simulink model "AeropendulumSoftRTBangBang"  (Simulink 7.9)
settings: Solver=FixedStepDiscrete  SolverMode=SingleTasking  StartTime=0.0  StopTime=60  RelTol=1e-3
PreLoadFcn:
  | u0=21;
  | Slope=80;
  | Clag=1;
  | Clead=1;
  | clagd=1;
  | clead=1;
InitFcn:
  | out = instrfind;
  | delete(out);
  | s = serial('COM5');
  | set(s,'BaudRate',19200);
  | set(s,'InputBufferSize',2);
  | fopen(s);
StartFcn:
  | fwrite(s,128,'uchar');
StopFcn:
  | fclose(s)
undefined symbols (not defined in the file or in its folder): fread, fwrite
libraries: simulink x5, cstblocks x2
Description:
  | AeroPendulum Controller
  | -Phase lead
  | -Phase lag
  | -Proportional control
  | 
  | All controllers working!
settings Model: Creator=Josh Gill  LastModifiedBy=Enikov  ExtModeEnableFloating=off  ExtModeTrigDuration=10000  ExtModeLogAll=off
settings DataIOCC: SaveOutput=off  SignalLogging=off  DSMLogging=off  SaveTime=off
settings DebuggingCC: FcnCallInpInsideContextMsg=Use local settings  StrictBusMsg=Warning
settings HardwareCC: ProdIntDivRoundTo=Zero  ProdEndianess=LittleEndian  ProdHWDeviceType=Generic->32-bit x86 compatible
settings RTWCC: SystemTargetFile=rtwin.tlc  TemplateMakefile=rtwin.tmf  Description=Real-Time Windows Target  ProcessScript=rtwin_make_rtw_hook  RTWCompilerOptimization=On
settings CodeAppCC: MaxIdLength=95
settings RTWinTargetCC: TargetLibSuffix=_rtwin.lib  TargetPreCompLibLocation=C:\Program Files\MATLAB\R2012a\toolbox\rtw\targets\rtwin\lib\win64  CodeReplacementLibrary=ANSI_C  CodeExecutionProfiling=off  PortableWordSizes=off  RTWinDir=C:/PROGRA~1/MATLAB/R2012a/toolbox/rtw/targets/rtwin  TargetArch=win64

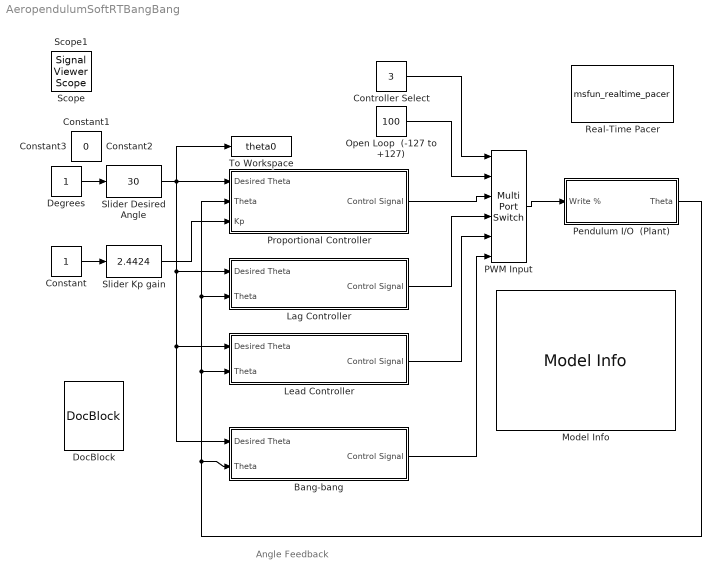
== system AeropendulumSoftRTBangBang ==
  note: Angle Feedback
  Bang-bang : Subsystem
  Constant : Constant
  Controller Select : Constant  Value=3
  Degrees : Constant
  DocBlock : simulink/Model-Wide Utilities/DocBlock  DocumentType=Text
  Lag Controller : Subsystem
  Lead Controller : Subsystem
  Model Info : simulink/Model-Wide Utilities/Model Info  InitialBlockCM=None  BlockCM=None  Frame=on  DisplayStringWithTags=|  HorizontalTextAlignment=Center  LeftAlignmentValue=0.5  SourceBlockDiagram=AeropendulumSoftRTBangBang  TagMaxNumber=20
      | %<Description>
      | --------------------------------------
      | %<ModifiedBy>
      | %<ModifiedDate>
      | %<ModelVersion>
  Open Loop  (-127 to +127) : Constant  Value=100
  PWM Input : MultiPortSwitch  Inputs=5  zeroidx=off
  Pendulum I/O  (Plant) : Subsystem
  Proportional Controller : Subsystem
  Real-Time Pacer : M-S-Function  FunctionName=msfun_realtime_pacer  Parameters=simTimePerRealTime  mask(RealTime_Pacer){simTimePerRealTime=1}
      mask prompts: simTimePerRealTime "Speedup (Simulation Time / Real Time):"
      mask help:
      | Slow down a simulation to track real (i.e., wall clock) elapsed time.
      |
      | "Speedup" specifies the ratio between simulation time and real time
      |  Speedup = N => N sec. of simulation time per sec. of real time
      |  Speedup can be fractional (e.g., 0.5, 1.3).
      |  Speedup = inf => allow simulation to run at full speed
      |
      | Click on the Help button for details.
      mask Help: web('realtime_pacer_help.html', '-helpbrowser')
      mask Display: fprintf('Real-Time Pacer\nSpeedup = %g', simTimePerRealTime)
  Slider Desired Angle : simulink/Math Operations/Slider Gain  low=0  gain=30  high=60
  Slider Kp gain : simulink/Math Operations/Slider Gain  low=0  gain=2.4424  high=5
  To Workspace : ToWorkspace  VariableName=theta0  SampleTime=-1
  Constant1 : Constant  IOType=siggen  Value=35
  Constant2 : Constant  IOType=siggen  Value=-20
  Constant3 : Constant  IOType=siggen  Value=0
  Scope : SignalViewerScope  IOType=viewer  RefreshTime=0.035000
  Scope1 : SignalViewerScope  IOType=viewer  ExtModeUploadOption=log  ZoomMode=yonly  LegendLocations="0.59858     0.75199     0.35106     0.12287"  RefreshTime=0.010417
      settings: TickLabels=on  ShowLegends=on  TimeRange=60  YMin=-50  YMax=140  SaveToWorkspace=on  MaxDataPoints=10000
  wires:
  Pendulum I/O  (Plant)/1(Theta) -> Proportional Controller/2(Theta), Lag Controller/2(Theta), Lead Controller/2(Theta), Bang-bang/2(Theta)
  PWM Input/1 -> Pendulum I/O  (Plant)/1(Write %)
  Open Loop  (-127 to +127)/1 -> PWM Input/2
  Proportional Controller/1(Control Signal) -> PWM Input/3
  Lag Controller/1(Control Signal) -> PWM Input/4
  Lead Controller/1(Control Signal) -> PWM Input/5
  Controller Select/1 -> PWM Input/1
  Slider Desired Angle/1 -> Proportional Controller/1(Desired Theta), To Workspace/1, Lag Controller/1(Desired Theta), Lead Controller/1(Desired Theta), Bang-bang/1(Desired Theta)
  Degrees/1 -> Slider Desired Angle/1
  Constant/1 -> Slider Kp gain/1
  Slider Kp gain/1 -> Proportional Controller/3(Kp)
  Bang-bang/1(Control Signal) -> PWM Input/6

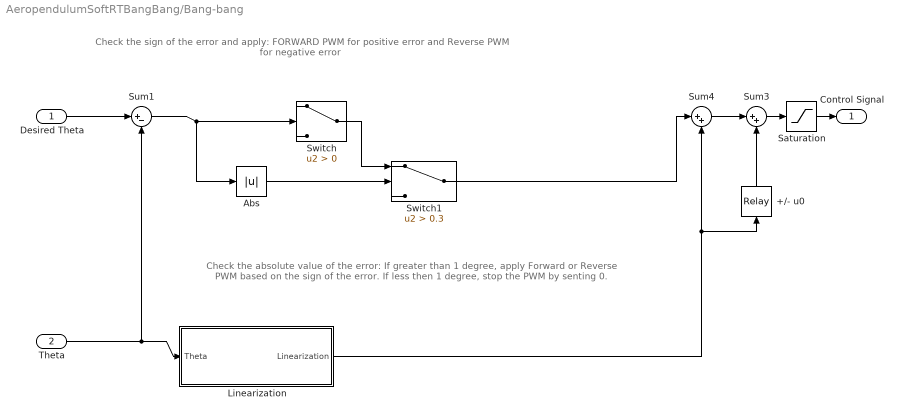
== system AeropendulumSoftRTBangBang/Bang-bang ==
  note: Check the absolute value of the error:
      | If greater than 1 degree,  apply
      | Forward or Reverse PWM
      | based on the sign of the error.
      |
      | If less then 1 degree,
      |  stop the PWM  by senting  0.
  note: Check the sign of the error and apply:
      |
      | FORWARD PWM for positive error
      | and
      | Reverse PWM for negative error
  Desired Theta : Inport
  Theta : Inport  Port=2
  +/- u0 : Relay  OffSwitchValue=-eps  OnOutputValue=u0
  Abs : Abs
  Linearization : Subsystem
  Saturation : Saturate  UpperLimit=127  LowerLimit=-127
  Sum1 : Sum  Inputs=|+-
  Sum3 : Sum  Inputs=|++
  Sum4 : Sum  Inputs=|++
  Switch : Switch  Criteria=u2 > Threshold
  Switch1 : Switch  Criteria=u2 > Threshold  Threshold=0.3
  Control Signal : Outport
  wires:
  Theta/1 -> Linearization/1(Theta), Sum1/2
  Desired Theta/1 -> Sum1/1
  Sum4/1 -> Sum3/1
  Saturation/1 -> Control Signal/1
  Linearization/1(Linearization) -> Sum4/2, +/- u0/1
  Sum1/1 -> Switch/2, Abs/1
  +/- u0/1 -> Sum3/2
  Sum3/1 -> Saturation/1
  Abs/1 -> Switch1/2
  Switch/1 -> Switch1/1
  Switch1/1 -> Sum4/1

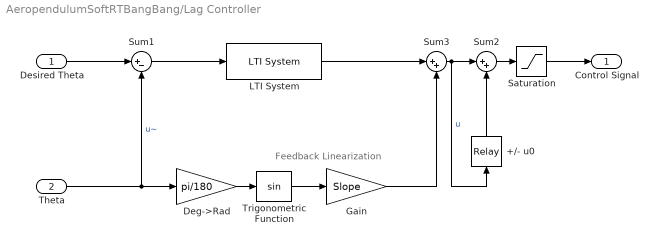
== system AeropendulumSoftRTBangBang/Lag Controller ==
  note: Feedback Linearization
  Desired Theta : Inport
  Theta : Inport  Port=2
  +/- u0 : Relay  OffSwitchValue=-eps  OnOutputValue=u0  OffOutputValue=-u0
  Deg->Rad : Gain  Gain=pi/180
  Gain : Gain  Gain=Slope
  LTI System : cstblocks/LTI System  sys=clagd  IC=[]
  Saturation : Saturate  UpperLimit=127  LowerLimit=-127
  Sum1 : Sum  Inputs=|+-
  Sum2 : Sum  Inputs=|++
  Sum3 : Sum  Inputs=|++
  Trigonometric Function : Trigonometry
  Control Signal : Outport
  wires:
  Desired Theta/1 -> Sum1/1
  Sum1/1 -> LTI System/1
  Saturation/1 -> Control Signal/1
  LTI System/1 -> Sum3/1
  Theta/1 -> Sum1/2, Deg->Rad/1  "u~"
  Sum3/1 -> +/- u0/1, Sum2/1  "u"
  Deg->Rad/1 -> Trigonometric Function/1
  Trigonometric Function/1 -> Gain/1
  Gain/1 -> Sum3/2
  +/- u0/1 -> Sum2/2
  Sum2/1 -> Saturation/1

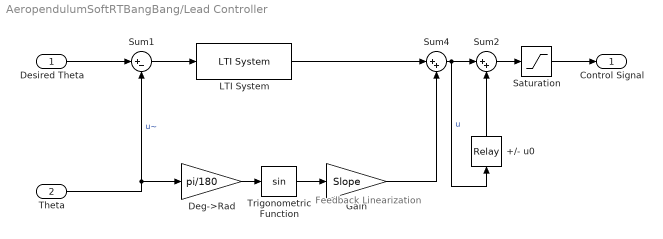
== system AeropendulumSoftRTBangBang/Lead Controller ==
  note: Feedback Linearization
  Desired Theta : Inport
  Theta : Inport  Port=2
  +/- u0 : Relay  OffSwitchValue=-eps  OnOutputValue=u0  OffOutputValue=-u0
  Deg->Rad : Gain  Gain=pi/180
  Gain : Gain  Gain=Slope
  LTI System : cstblocks/LTI System  sys=clead  IC=[]
  Saturation : Saturate  UpperLimit=127  LowerLimit=-127
  Sum1 : Sum  Inputs=|+-
  Sum2 : Sum  Inputs=|++
  Sum4 : Sum  Inputs=|++
  Trigonometric Function : Trigonometry
  Control Signal : Outport
  wires:
  Desired Theta/1 -> Sum1/1
  Sum4/1 -> +/- u0/1, Sum2/1  "u"
  Saturation/1 -> Control Signal/1
  Sum1/1 -> LTI System/1
  LTI System/1 -> Sum4/1
  Theta/1 -> Sum1/2, Deg->Rad/1  "u~"
  Deg->Rad/1 -> Trigonometric Function/1
  Trigonometric Function/1 -> Gain/1
  Gain/1 -> Sum4/2
  +/- u0/1 -> Sum2/2
  Sum2/1 -> Saturation/1

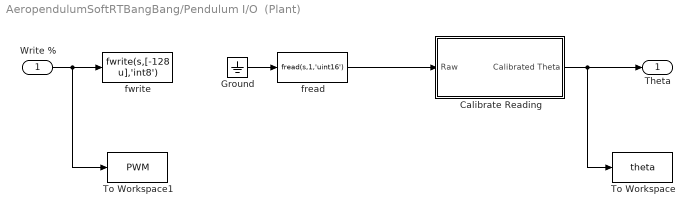
== system AeropendulumSoftRTBangBang/Pendulum I/O  (Plant) ==
  Write % : Inport
  Calibrate Reading : Subsystem
  Ground : Ground
  To Workspace : ToWorkspace  VariableName=theta  SampleTime=-1
  To Workspace1 : ToWorkspace  VariableName=PWM  SampleTime=-1
  fread : MATLABFcn  MATLABFcn=fread(s,1,'uint16')  OutputDimensions=1  OutputSignalType=real  Output1D=off  SampleTime=0.01
  fwrite : MATLABFcn  MATLABFcn=fwrite(s,[-128 u],'int8')  OutputDimensions=0  OutputSignalType=real  SampleTime=0.01
  Theta : Outport
  wires:
  Write %/1 -> To Workspace1/1, fwrite/1
  Calibrate Reading/1(Calibrated Theta) -> Theta/1, To Workspace/1
  fread/1 -> Calibrate Reading/1(Raw)
  Ground/1 -> fread/1

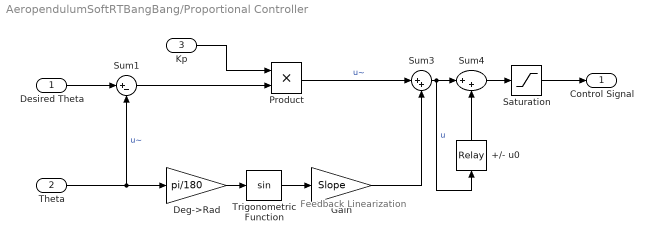
== system AeropendulumSoftRTBangBang/Proportional Controller ==
  note: Feedback Linearization
  Desired Theta : Inport
  Theta : Inport  Port=2
  Kp : Inport  Port=3
  +/- u0 : Relay  OffSwitchValue=-eps  OnOutputValue=u0  OffOutputValue=-u0
  Deg->Rad : Gain  Gain=pi/180
  Gain : Gain  Gain=Slope
  Product : Product  RndMeth=Zero
  Saturation : Saturate  UpperLimit=127  LowerLimit=-127
  Sum1 : Sum  Inputs=|+-
  Sum3 : Sum  Inputs=|++
  Sum4 : Sum  Inputs=|++
  Trigonometric Function : Trigonometry
  Control Signal : Outport
  wires:
  Theta/1 -> Sum1/2, Deg->Rad/1  "u~"
  Desired Theta/1 -> Sum1/1
  Sum1/1 -> Product/2
  Saturation/1 -> Control Signal/1
  Product/1 -> Sum3/1  "u~"
  Deg->Rad/1 -> Trigonometric Function/1
  Trigonometric Function/1 -> Gain/1
  Gain/1 -> Sum3/2
  Kp/1 -> Product/1
  Sum4/1 -> Saturation/1
  Sum3/1 -> Sum4/1, +/- u0/1  "u"
  +/- u0/1 -> Sum4/2

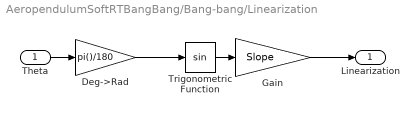
== system AeropendulumSoftRTBangBang/Bang-bang/Linearization ==
  Theta : Inport
  Deg->Rad : Gain  Gain=pi()/180
  Gain : Gain  Gain=Slope
  Trigonometric Function : Trigonometry
  Linearization : Outport
  wires:
  Trigonometric Function/1 -> Gain/1
  Deg->Rad/1 -> Trigonometric Function/1
  Theta/1 -> Deg->Rad/1
  Gain/1 -> Linearization/1

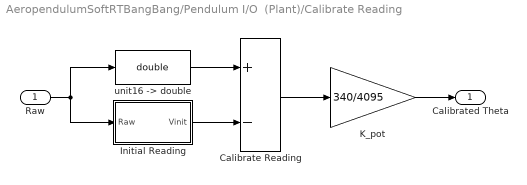
== system AeropendulumSoftRTBangBang/Pendulum I/O  (Plant)/Calibrate Reading ==
  Raw : Inport
  Calibrate Reading : Sum  Inputs=+-
  Initial Reading : Subsystem
  K_pot : Gain  Gain=340/4095  OutDataTypeStr=Inherit: Inherit via back propagation  SaturateOnIntegerOverflow=on
  "unit16 -> double" : DataTypeConversion  OutDataTypeStr=double
  Calibrated Theta : Outport
  wires:
  "unit16 -> double"/1 -> Calibrate Reading/1
  K_pot/1 -> Calibrated Theta/1
  Calibrate Reading/1 -> K_pot/1
  Raw/1 -> "unit16 -> double"/1, Initial Reading/1(Raw)
  Initial Reading/1(Vinit) -> Calibrate Reading/2

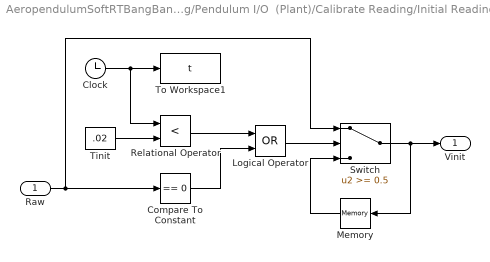
== system AeropendulumSoftRTBangBang/Pendulum I/O  (Plant)/Calibrate Reading/Initial Reading ==
  Raw : Inport
  Clock : Clock
  Compare To Constant : simulink/Logic and Bit Operations/Compare To Constant  relop===  const=0  OutDataTypeStr=boolean
  Logical Operator : Logic  Operator=OR  AllPortsSameDT=off  OutDataTypeStr=boolean
  Memory : Memory  InheritSampleTime=on  LinearizeAsDelay=on
  Relational Operator : RelationalOperator  Operator=<  OutDataTypeStr=boolean
  Switch : Switch  Threshold=0.5
  Tinit : Constant  Value=.02
  To Workspace1 : ToWorkspace  VariableName=t  SampleTime=-1
  Vinit : Outport
  wires:
  Memory/1 -> Switch/3
  Switch/1 -> Vinit/1, Memory/1
  Logical Operator/1 -> Switch/2
  Compare To Constant/1 -> Logical Operator/2
  Relational Operator/1 -> Logical Operator/1
  Raw/1 -> Switch/1, Compare To Constant/1
  Tinit/1 -> Relational Operator/2
  Clock/1 -> Relational Operator/1, To Workspace1/1
